simulink model "laboC3_Vlsi"  (R2021b)
settings: Solver=VariableStepAuto  StartTime=0.0  StopTime=100e-6  RelTol=1e-3
libraries: hdlBasic x75, xbsIndex_r4 x1
settings Model: Creator=Darryl  LastModifiedBy=Darryl

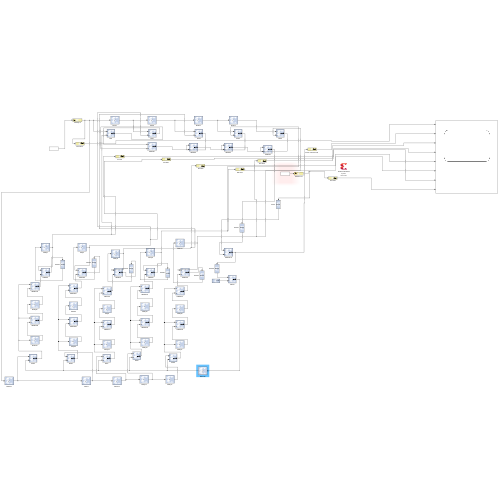
[thumbnail: Simulink's stored preview of the top-level diagram]
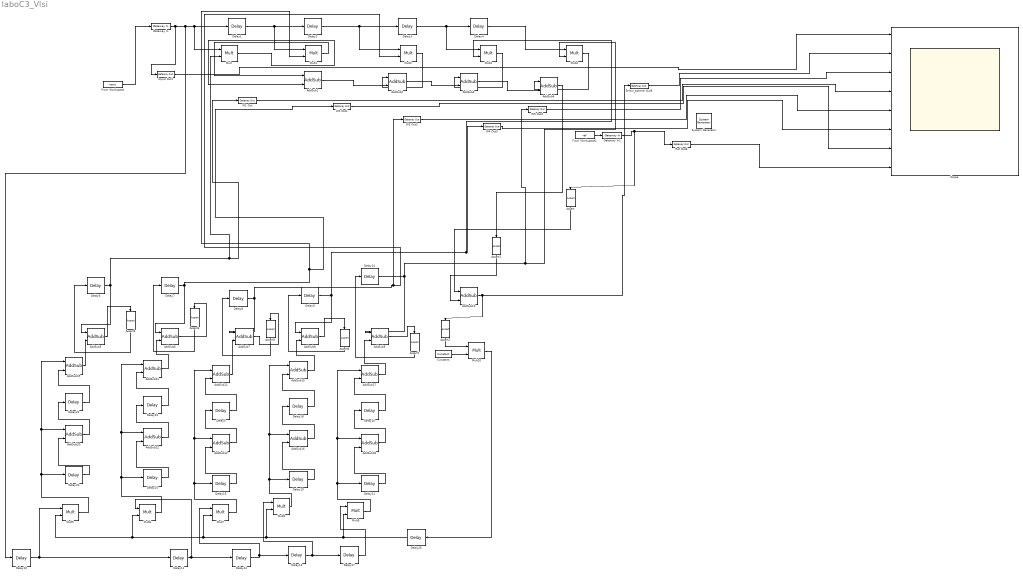
== system laboC3_Vlsi ==
  " System Generator" : xbsIndex_r4/ System Generator  Tag=genX  xilinxfamily=kintex7  part=xc7k325t  speed=-3  package=fbg676  synthesis_tool=Vivado  clock_wrapper=Clock Enables  directory=./netlist  proj_type=Vivado  Synth_file=Vivado Synthesis Defaults  Impl_file=Vivado Implementation Defaults  testbench=off  simulink_period=1/20e6  sysclk_period=50  dcm_input_clock_period=10  incr_netlist=off  trim_vbits=Everywhere in SubSystem  dbl_ovrd=According to Block Masks  core_generation=According to Block Masks  run_coregen=off  deprecated_control=off  eval_field=0  block_type=sysgen
  AddSub{1..9,11..12,15..22} (19 alike) : hdlBasic/AddSub  mode=Addition  use_carryin=off  use_carryout=off  en=off  latency=0  precision=User Defined  arith_type="Signed  (2's comp)"  n_bits=16  bin_pt=14  quantization=Truncate  overflow=Wrap  use_behavioral_HDL=off  hw_selection=Fabric  pipelined=off  XmcBlockStatus=1  maskContainerNames=tabcontainer1  block_type=addsub  block_config=sysgen:Addsub_config
  AddSub10 : hdlBasic/AddSub  mode=Subtraction  use_carryin=off  use_carryout=off  en=off  latency=0  precision=User Defined  arith_type="Signed  (2's comp)"  n_bits=16  bin_pt=14  quantization=Truncate  overflow=Wrap  use_behavioral_HDL=off  hw_selection=Fabric  pipelined=off  XmcBlockStatus=1  maskContainerNames=tabcontainer1  block_type=addsub  block_config=sysgen:Addsub_config
  Assert{,1..7} (8 alike) : hdlBasic/Assert  assert_type=on  type_source=Explicitly  gui_display_data_type=Fixed-point  arith_type=Signed (2's comp)  n_bits=16  bin_pt=14  preci_type=Single  exp_width=8  frac_width=24  assert_rate=on  rate_source=Explicitly  period=1/20e6  output_port=on  XmcBlockStatus=1  maskContainerNames=group1  block_type=assert  block_config=sysgen:assert_config
  Constant : hdlBasic/Constant  const=0.25  gui_display_data_type=Fixed-point  arith_type=Signed (2's comp)  n_bits=16  bin_pt=14  preci_type=Single  exp_width=8  frac_width=24  explicit_period=off  period=1  XmcBlockStatus=1  maskContainerNames=tabcontainer1  block_type=constant  block_config=sysgen:Constant_config
  Delay{1..5,11..13,15,17..25} (18 alike) : hdlBasic/Delay  rst=off  en=off  latency=1  reg_retiming=off  XmcBlockStatus=1  maskContainerNames=group1  block_type=delay  block_config=sysgen:Delay_config
  Delay10 : hdlBasic/Delay  rst=off  en=off  latency=5  reg_retiming=off  XmcBlockStatus=1  maskContainerNames=group1  block_type=delay  block_config=sysgen:Delay_config
  Delay{6..9,14} (5 alike) : hdlBasic/Delay  rst=off  en=off  latency=3  reg_retiming=off  XmcBlockStatus=1  maskContainerNames=group1  block_type=delay  block_config=sysgen:Delay_config
  Delay26 : hdlBasic/Delay  rst=off  en=off  latency=5  reg_retiming=off  XmcBlockStatus=1  maskContainerNames=group1  block_type=delay  block_config=sysgen:Delay_config
  Erreur_estimer Out5 : hdlBasic/Gateway Out  inherit_from_input=off  hdl_port=on  rows=1  columns=1  UseAsDAC=off  DACChannel='1'  interface=None  automatic_assignment=on  address_offset=hex2dec('00')  intf_name=''  intf_description=''  timing_constraint=None  locs_specified=off  LOCs={}  io_standard={}  XmcBlockStatus=1  maskContainerNames=group4  block_type=gatewayout  block_config=sysgen:gateway_out_config  block_width_w=590  block_height_w=620  block_width=620  block_height=750
  From Workspace : FromWorkspace  VariableName=input
  From Workspace1 : FromWorkspace  VariableName=ref
  Gateway In : hdlBasic/Gateway In  gui_display_data_type=Fixed-point  arith_type=Signed (2's comp)  n_bits=16  bin_pt=14  preci_type=Single  exp_width=8  frac_width=24  rows=1  columns=1  quantization="Round  (unbiased: +/- Inf)"  overflow=Saturate  period=1/20e6  UseAsADC=off  ADCChannel='1'  interface=None  automatic_assignment=on  address_offset=hex2dec('00')  intf_name=''  intf_description=''  default_value=0  timing_constraint=None  locs_specified=off  LOCs={}  io_standard={}  inherit_from_input=off  hdl_port=on  XmcBlockStatus=1  maskContainerNames=group4  block_type=gatewayin  block_config=sysgen:gateway_in_config  block_width_w=590  block_height_w=620  block_width=640  block_height=850
  Gateway In1 : hdlBasic/Gateway In  gui_display_data_type=Fixed-point  arith_type=Signed (2's comp)  n_bits=16  bin_pt=14  preci_type=Single  exp_width=8  frac_width=24  rows=1  columns=1  quantization="Round  (unbiased: +/- Inf)"  overflow=Saturate  period=1/20e6  UseAsADC=off  ADCChannel='1'  interface=None  automatic_assignment=on  address_offset=hex2dec('00')  intf_name=''  intf_description=''  default_value=0  timing_constraint=None  locs_specified=off  LOCs={}  io_standard={}  inherit_from_input=off  hdl_port=on  XmcBlockStatus=1  maskContainerNames=group4  block_type=gatewayin  block_config=sysgen:gateway_in_config  block_width_w=590  block_height_w=620  block_width=640  block_height=850
  Mult{,1..10} (11 alike) : hdlBasic/Mult  precision=User Defined  arith_type="Signed  (2's comp)"  n_bits=16  bin_pt=14  quantization=Truncate  overflow=Wrap  en=off  latency=0  use_behavioral_HDL=off  opt=Speed  use_embedded=on  optimum_pipeline=off  pipeline=on  use_rpm=on  placement_style=Triangular  XmcBlockStatus=1  maskContainerNames=group1  block_type=mult  block_config=sysgen:Mult_config
  Ref Out6 : hdlBasic/Gateway Out  inherit_from_input=off  hdl_port=on  rows=1  columns=1  UseAsDAC=off  DACChannel='1'  interface=None  automatic_assignment=on  address_offset=hex2dec('00')  intf_name=''  intf_description=''  timing_constraint=None  locs_specified=off  LOCs={}  io_standard={}  XmcBlockStatus=1  maskContainerNames=group4  block_type=gatewayout  block_config=sysgen:gateway_out_config  block_width_w=590  block_height_w=620  block_width=620  block_height=750
  Scope : Scope  NumInputPorts=8
  W1 Out : hdlBasic/Gateway Out  inherit_from_input=off  hdl_port=on  rows=1  columns=1  UseAsDAC=off  DACChannel='1'  interface=None  automatic_assignment=on  address_offset=hex2dec('00')  intf_name=''  intf_description=''  timing_constraint=None  locs_specified=off  LOCs={}  io_standard={}  XmcBlockStatus=1  maskContainerNames=group4  block_type=gatewayout  block_config=sysgen:gateway_out_config  block_width_w=590  block_height_w=620  block_width=620  block_height=750
  W2 Out1 : hdlBasic/Gateway Out  inherit_from_input=off  hdl_port=on  rows=1  columns=1  UseAsDAC=off  DACChannel='1'  interface=None  automatic_assignment=on  address_offset=hex2dec('00')  intf_name=''  intf_description=''  timing_constraint=None  locs_specified=off  LOCs={}  io_standard={}  XmcBlockStatus=1  maskContainerNames=group4  block_type=gatewayout  block_config=sysgen:gateway_out_config  block_width_w=590  block_height_w=620  block_width=620  block_height=750
  W3 Out2 : hdlBasic/Gateway Out  inherit_from_input=off  hdl_port=on  rows=1  columns=1  UseAsDAC=off  DACChannel='1'  interface=None  automatic_assignment=on  address_offset=hex2dec('00')  intf_name=''  intf_description=''  timing_constraint=None  locs_specified=off  LOCs={}  io_standard={}  XmcBlockStatus=1  maskContainerNames=group4  block_type=gatewayout  block_config=sysgen:gateway_out_config  block_width_w=590  block_height_w=620  block_width=620  block_height=750
  W4 Out3 : hdlBasic/Gateway Out  inherit_from_input=off  hdl_port=on  rows=1  columns=1  UseAsDAC=off  DACChannel='1'  interface=None  automatic_assignment=on  address_offset=hex2dec('00')  intf_name=''  intf_description=''  timing_constraint=None  locs_specified=off  LOCs={}  io_standard={}  XmcBlockStatus=1  maskContainerNames=group4  block_type=gatewayout  block_config=sysgen:gateway_out_config  block_width_w=590  block_height_w=620  block_width=620  block_height=750
  W5 Out4 : hdlBasic/Gateway Out  inherit_from_input=off  hdl_port=on  rows=1  columns=1  UseAsDAC=off  DACChannel='1'  interface=None  automatic_assignment=on  address_offset=hex2dec('00')  intf_name=''  intf_description=''  timing_constraint=None  locs_specified=off  LOCs={}  io_standard={}  XmcBlockStatus=1  maskContainerNames=group4  block_type=gatewayout  block_config=sysgen:gateway_out_config  block_width_w=590  block_height_w=620  block_width=620  block_height=750
  imput Out1 : hdlBasic/Gateway Out  inherit_from_input=off  hdl_port=on  rows=1  columns=1  UseAsDAC=off  DACChannel='1'  interface=None  automatic_assignment=on  address_offset=hex2dec('00')  intf_name=''  intf_description=''  timing_constraint=None  locs_specified=off  LOCs={}  io_standard={}  XmcBlockStatus=1  maskContainerNames=group4  block_type=gatewayout  block_config=sysgen:gateway_out_config  block_width_w=590  block_height_w=620  block_width=620  block_height=750
  wires:
  imput Out1/1 -> Scope/1
  Erreur_estimer Out5/1 -> Scope/2
  W5 Out4/1 -> Scope/3
  W1 Out/1 -> Scope/4
  W3 Out2/1 -> Scope/5
  W4 Out3/1 -> Scope/6
  W2 Out1/1 -> Scope/7
  Ref Out6/1 -> Scope/8
  From Workspace/1 -> Gateway In/1
  Delay4/1 -> Mult4/1
  Mult1/1 -> AddSub1/1
  Delay2/1 -> Mult2/1, Delay3/1
  Mult3/1 -> AddSub3/1
  Mult/1 -> AddSub1/2
  AddSub3/1 -> AddSub4/2
  Mult4/1 -> AddSub4/1
  Delay1/1 -> Mult1/1, Delay2/1
  Delay8/1 -> Mult2/2, W3 Out2/1, AddSub7/1
  Delay3/1 -> Mult3/1, Delay4/1
  From Workspace1/1 -> Gateway In1/1
  Delay7/1 -> AddSub6/1, W2 Out1/1, Mult1/2
  Mult2/1 -> AddSub2/1
  Delay14/1 -> AddSub9/1, Mult4/2, W5 Out4/1
  Delay6/1 -> AddSub5/1, W1 Out/1, Mult/2
  AddSub10/1 -> Assert2/1, Erreur_estimer Out5/1
  AddSub2/1 -> AddSub3/2
  Delay9/1 -> W4 Out3/1, Mult3/2, AddSub8/1
  AddSub1/1 -> AddSub2/2
  AddSub17/1 -> AddSub9/2
  Mult9/1 -> Delay21/1, AddSub17/1, AddSub18/1
  AddSub18/1 -> Delay20/1
  Delay21/1 -> AddSub18/2
  Delay20/1 -> AddSub17/2
  AddSub15/1 -> AddSub8/2
  Mult8/1 -> Delay19/1, AddSub16/1, AddSub15/1
  AddSub16/1 -> Delay18/1
  Delay19/1 -> AddSub16/2
  Delay18/1 -> AddSub15/2
  AddSub11/1 -> AddSub7/2
  Mult7/1 -> Delay15/1, AddSub11/1, AddSub12/1
  AddSub19/1 -> AddSub5/2
  AddSub21/1 -> AddSub6/2
  Mult6/1 -> Delay25/1, AddSub21/1, AddSub22/1
  AddSub12/1 -> Delay5/1
  Delay15/1 -> AddSub12/2
  Delay5/1 -> AddSub11/2
  Mult5/1 -> Delay23/1, AddSub19/1, AddSub20/1
  Delay24/1 -> AddSub21/2
  AddSub22/1 -> Delay24/1
  Delay25/1 -> AddSub22/2
  Delay23/1 -> AddSub20/2
  AddSub20/1 -> Delay22/1
  Delay22/1 -> AddSub19/2
  Constant/1 -> Mult10/2
  Delay13/1 -> Mult8/1, Delay17/1
  Mult10/1 -> Delay26/1
  Delay12/1 -> Delay13/1, Mult7/1
  Gateway In/1 -> imput Out1/1, Delay10/1, Mult/1, Delay1/1
  Gateway In1/1 -> Assert/1, Ref Out6/1
  Delay10/1 -> Mult5/1, Delay11/1
  Delay11/1 -> Mult6/1, Delay12/1
  Delay26/1 -> Mult9/2, Mult8/2, Mult7/2, Mult6/2, Mult5/2
  Delay17/1 -> Mult9/1
  Assert/1 -> AddSub10/1
  Assert1/1 -> AddSub10/2
  AddSub4/1 -> Assert1/1
  Assert2/1 -> Mult10/1
  AddSub6/1 -> Assert3/1
  Assert3/1 -> Delay7/1
  AddSub5/1 -> Assert4/1
  Assert4/1 -> Delay6/1
  AddSub7/1 -> Assert5/1
  Assert5/1 -> Delay8/1
  AddSub8/1 -> Assert6/1
  Assert6/1 -> Delay9/1
  Assert7/1 -> Delay14/1
  AddSub9/1 -> Assert7/1
